simulink model "sim_tp_matlab_r2016a"  (Simulink 8.7)
settings: Solver=VariableStepAuto  SolverMode=SingleTasking  StartTime=0.0  StopTime=10*pi  RelTol=1e-7  AbsTol=1e-7
values from neighbouring files (symbols this model uses):
  Te = s.DialogPrm(1).Data    [sf_mpc_controller.m]
settings Model: Creator=danes  LastModifiedBy=danes
settings DataIOCC: LimitDataPoints=off  SaveFormat=Dataset  ReturnWorkspaceOutputs=on
settings DebuggingCC: UnderspecifiedInitializationDetection=Simplified  MergeDetectMultiDrivingBlocksExec=error  SFUnexpectedBacktrackingDiag=error  SFNoUnconditionalDefaultTransitionDiag=error
settings HardwareCC: ProdBitPerPointer=64  ProdLargestAtomicFloat=Float  ProdIntDivRoundTo=Zero  ProdEndianess=LittleEndian  ProdWordSize=64  ProdHWDeviceType=Intel->x86-64 (Windows64)
settings ModelReferenceCC: PropagateSignalLabelsOutOfModel=on
settings SFSimCC: SimUseLocalCustomCode=on
settings RTWCC: RTWUseLocalCustomCode=on
settings GRTTargetCC: TargetLangStandard=C99 (ISO)  GeneratePreprocessorConditionals=Use local settings
settings ConfigComp: CovMetricSettings=dwe  CovHtmlReporting=off  CovSaveCumulativeToWorkspaceVar=off  CovSaveSingleToWorkspaceVar=off  CovModelRefEnable=off  CovExternalEMLEnable=on

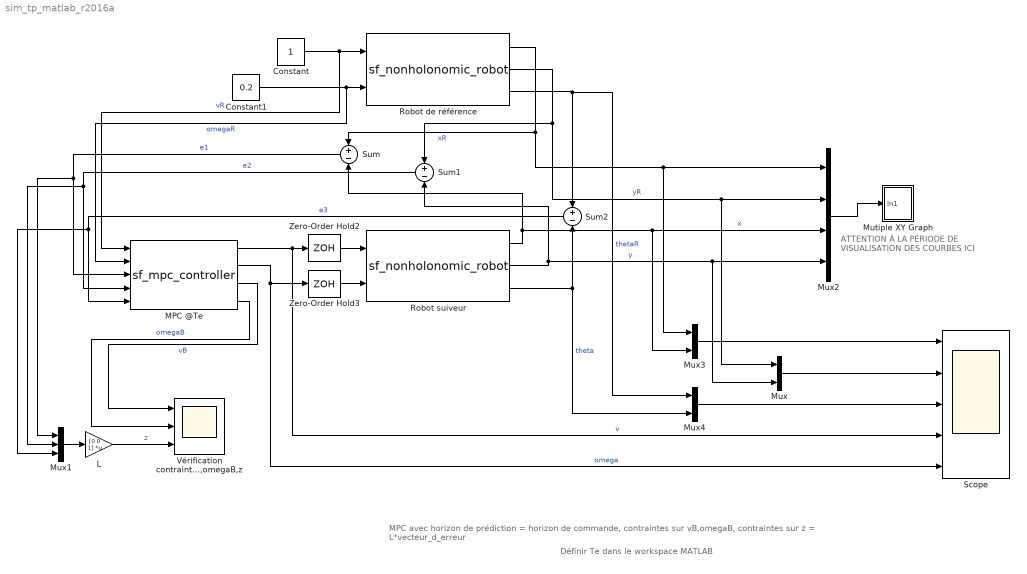
== system sim_tp_matlab_r2016a ==
  note: ATTENTION À LA PÉRIODE
      | DE VISUALISATION DES COURBES
      | ICI
  note: MPC avec horizon de prédiction = horizon de commande, contraintes sur vB,omegaB, contraintes sur z = L*vecteur_d_erreur
  note: Définir Te dans le workspace MATLAB
  Constant : Constant
  Constant1 : Constant  Value=0.2
  L : Gain  Gain=[0 0 1]  Multiplication=Matrix(K*u)
  MPC @Te : M-S-Function  FunctionName=sf_mpc_controller  Parameters=Te Np Nu L  mask{Te=Te, Np=100, Nu=100, L=[0 0 1]}
      mask prompts: Te "Sampling Period"; Np "Prediction Horizon"; Nu "Control Horizon"; L "L matrix such that z = L*e"
  Mutiple XY Graph : Subsystem  mask(Mutiple XY Graph){number_of_trajectories=2, axis_limits=[-6 6 -2 12], sample_time=min(20*Te,0.25)}
      mask prompts: number_of_trajectories "Number of Trajectories"; axis_limits "Axis Limits"; sample_time "Sample Time"
      mask Display: plot([.05 .95 .95 .05 .05],[.45 .45 .95 .95 .45], 0.5+cos(0:0.1:2*pi)*0.3,0.7+sin(0:0.1:2*pi)*0.2)
  Mux : Mux  Inputs=2
  Mux1 : Mux  Inputs=3
  Mux2 : Mux
  Mux3 : Mux  Inputs=2
  Mux4 : Mux  Inputs=2
  Robot de référence : M-S-Function  FunctionName=sf_nonholonomic_robot  Parameters=X0  mask{X0=[0;0;0];}
      mask prompts: X0 "Initial state (3x1)"
  Robot suiveur : M-S-Function  FunctionName=sf_nonholonomic_robot  Parameters=X0  mask{X0=[-1 ; -1 ; pi/3]}
      mask prompts: X0 "Initial state (3x1)"
  Scope : Scope  NumInputPorts=5
  Sum : Sum  Inputs=+|-
  Sum1 : Sum  Inputs=+|-
  Sum2 : Sum  Inputs=+|-
  Vérification contraintes sur vB,omegaB,z : Scope  NumInputPorts=3
  Zero-Order Hold2 : ZeroOrderHold  SampleTime=Te
  Zero-Order Hold3 : ZeroOrderHold  SampleTime=Te
  wires:
  Constant/1 -> Robot de référence/1, MPC @Te/1  "vR"
  Robot de référence/1 -> Mux3/1, Mux2/1, Sum/1  "xR"
  Robot de référence/2 -> Mux/1, Mux2/2, Sum1/1  "yR"
  MPC @Te/1 -> Scope/4, Zero-Order Hold2/1  "v"
  MPC @Te/2 -> Scope/5, Zero-Order Hold3/1  "omega"
  Robot suiveur/1 -> Mux3/2, Mux2/3, Sum/2  "x"
  Robot suiveur/2 -> Mux/2, Mux2/4, Sum1/2  "y"
  Robot suiveur/3 -> Mux4/2, Sum2/2  "theta"
  Sum/1 -> Mux1/1, MPC @Te/3  "e1"
  Sum1/1 -> Mux1/2, MPC @Te/4  "e2"
  Robot de référence/3 -> Mux4/1, Sum2/1  "thetaR"
  Sum2/1 -> Mux1/3, MPC @Te/5  "e3"
  Mux2/1 -> Mutiple XY Graph/1(In1)
  Mux3/1 -> Scope/1
  Mux/1 -> Scope/2
  Mux4/1 -> Scope/3
  Constant1/1 -> MPC @Te/2, Robot de référence/2  "omegaR"
  MPC @Te/3 -> Vérification contraintes sur vB,omegaB,z/1  "vB"
  MPC @Te/4 -> Vérification contraintes sur vB,omegaB,z/2  "omegaB"
  Mux1/1 -> L/1
  L/1 -> Vérification contraintes sur vB,omegaB,z/3  "z"
  Zero-Order Hold3/1 -> Robot suiveur/2
  Zero-Order Hold2/1 -> Robot suiveur/1

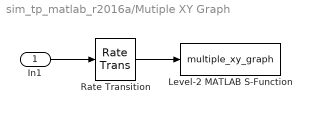
== system sim_tp_matlab_r2016a/Mutiple XY Graph ==
  In1 : Inport
  Level-2 MATLAB S-Function : M-S-Function  FunctionName=multiple_xy_graph  Parameters=number_of_trajectories,axis_limits
  Rate Transition : RateTransition  OutPortSampleTime=sample_time
  wires:
  Rate Transition/1 -> Level-2 MATLAB S-Function/1
  In1/1 -> Rate Transition/1
